simulink model "PTC_CI_L_Exp_20211"  (R2020b)
settings: Solver=VariableStepAuto  StartTime=0.0  StopTime=0.99  FixedStep=1e-6  MaxStep=1e-5  RelTol=1e-6
settings Model: Creator=Amir  LastModifiedBy=Amir
settings DataIOCC: ReturnWorkspaceOutputs=off

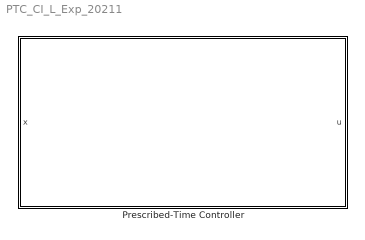
== system PTC_CI_L_Exp_20211 ==
  Prescribed-Time Controller : Subsystem  mask(Prescribed-Time Control for Normal form Systems - Version: PTC.CI.L.Exp.2021-1){n=1, tau=1, c=-1, alpha=1e-1}
      mask prompts: n "System dimension (n):"; tau "Convergence time (tau):"; c "Vector of control gains (c):"; alpha "Mapping coefficient (alpha):"
      mask Help:
      | This simulink block obtains a prescribed-time control for 'n' dimensional normal form systems (as perturbed chain of integrators):
      | 
      | dx1/dt=x2
      | dx2/dt=x3
      | .
      | .
      | .
      | dxn/dt=u+f(x)
      | 
      | where x=[x1;x2;...;xn] is a n-dimensional vector.
      | 
      | The input variables are:
      | 
      | n: The system dimension (or equivalently, order of the differential equation).
      | 
      | tau: The desired convergence time at which x=0 is reached.
      | 
      | c: n-dimensional vector of control gains.
      | 
      | alpha: A small enough positive mapping coefficient.
      mask DialogControl DescGroupVar Prompt: Main
      mask DialogControl DescTextVar Prompt: This block obtains a time-varying controller for a chain of integrators such that the convergence occurs at an arbitrary finite time 't=tau'. The response of the system would be globally triangularly stable if some conditions are hold.
      mask DialogControl Container7 Prompt: Parameters
      mask DialogControl Container7_copy Prompt: More
      mask DialogControl Control2 Prompt: For updated versions, other versions of prescribed-time control, and more stuff, refer to the following link:
      mask DialogControl Control3 Prompt: https://github.com/a-shakouri
      mask DialogControl Control3 Callback: web https://github.com/a-shakouri
      mask Display:
      | color('red');
      | disp('Prescribed-Time Control\n for Chain of Integrators\n\n Version: PTC.CI.L.Exp.2021-1')
      | color('blue');
      | port_label('output',1,'controller (u)','texmode','on');
      | port_label('input',1,'state vector (x)','texmode','on');

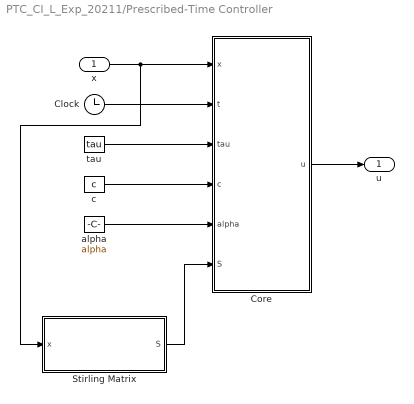
== system PTC_CI_L_Exp_20211/Prescribed-Time Controller ==
  x : Inport
  Clock : Clock
  Core : MATLAB Function  TreatAsAtomicUnit=on
  Stirling Matrix : MATLAB Function  TreatAsAtomicUnit=on
  alpha : Constant  Value=alpha
  c : Constant  Value=c
  tau : Constant  Value=tau
  u : Outport
  wires:
  tau/1 -> Core/3(tau)
  Clock/1 -> Core/2(t)
  c/1 -> Core/4(c)
  alpha/1 -> Core/5(alpha)
  x/1 -> Stirling Matrix/1(x), Core/1(x)
  Core/1(u) -> u/1
  Stirling Matrix/1(S) -> Core/6(S)

== matlab function PTC_CI_L_Exp_20211/Prescribed-Time Controller/Stirling Matrix ==
  data: x input size=[n 1]; S output size=[n n]
function S = Stirling_gen(x)

n=length(x);

S=zeros(n,n);

for i=1:n
    
    for j=1:n
        
        if i>=j
            
            m=0;

            for l=0:j-1
    
                sum=1/factorial(j-1)*(-1)^l*(factorial(j-1)/(factorial(l)*factorial(j-1-l)))*(j-1-l)^(i-1);
                
                m=m+sum;
                
            end
            
            S(i,j)=m;
            
        end
        
    end
    
end

== matlab function PTC_CI_L_Exp_20211/Prescribed-Time Controller/Core ==
  data: x input size=[n 1]; u output size=[1 1]; t input size=[1 1]; tau input size=[1 1]; c input size=[n 1]; alpha input size=[1 1]; S input size=[n n]
function u = PTC_gen(x,t,tau,c,alpha,S)

n=length(x);

u1=c(1)*x(1)/(alpha*(tau-t))^n;

u2=0;

for j=2:n
    
    u2in=0;
    
    for i=2:j
        
        u2in=u2in+S(j,i)*((-1)^(j-i)*x(i))/(tau-t)^(n-i+1);
        
    end
    
    u2=u2+c(j)/alpha^(n-j+1)*u2in;
    
end

u3=0;

for i=2:n
    
    u3=u3-S(n-1,i)*(-1)^(n-i+1)*x(i)/(tau-t)^(n-i+1);
    
end

u=u1+u2+u3;

% u=c'*x;
